simulink model "pwmoutput_exec"  (Simulink 3.00)
libraries: execlib x5

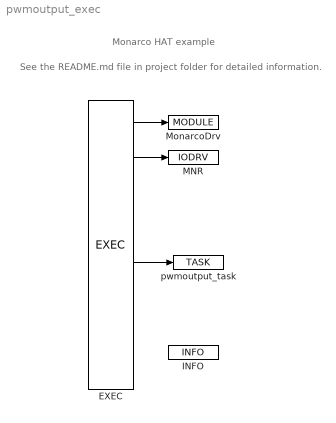
== system pwmoutput_exec ==
  note: See the README.md file in project
      | folder for detailed information.
  note: Monarco HAT example
  EXEC : execlib/EXEC  target=Generic target device  tick=0.01  ntick0=2  ntick1=50  ntick2=100  ntick3=1200  pri0=5  pri1=9  pri2=13  pri3=18
  INFO : execlib/INFO  Title=Monarco HAT - PWM output  Author=REX Controls s.r.o.  Description=Using PWM outputs of the Monarco HAT
  MNR : execlib/IODRV  module=MonarcoDrv  classname=MonarcoHatDrv  cfgname=monarcohat.rio  factor=1  stack=10240  pri=3  timer=off
  MonarcoDrv : execlib/MODULE
  pwmoutput_task : execlib/TASK  factor=1  start=0  stop=1  stack=10240  MDLOPEN=on
  wires:
  EXEC/1 -> MonarcoDrv/1
  EXEC/2 -> MNR/1
  EXEC/5 -> pwmoutput_task/1
